simulink model "serial_plot_v1"  (R2019a)
settings: Solver=VariableStepAuto  StartTime=0.0  StopTime=inf  RelTol=1e-3
libraries: instrumentlib x2
settings Model: Creator=facuolmed_o  LastModifiedBy=facuolmed_o

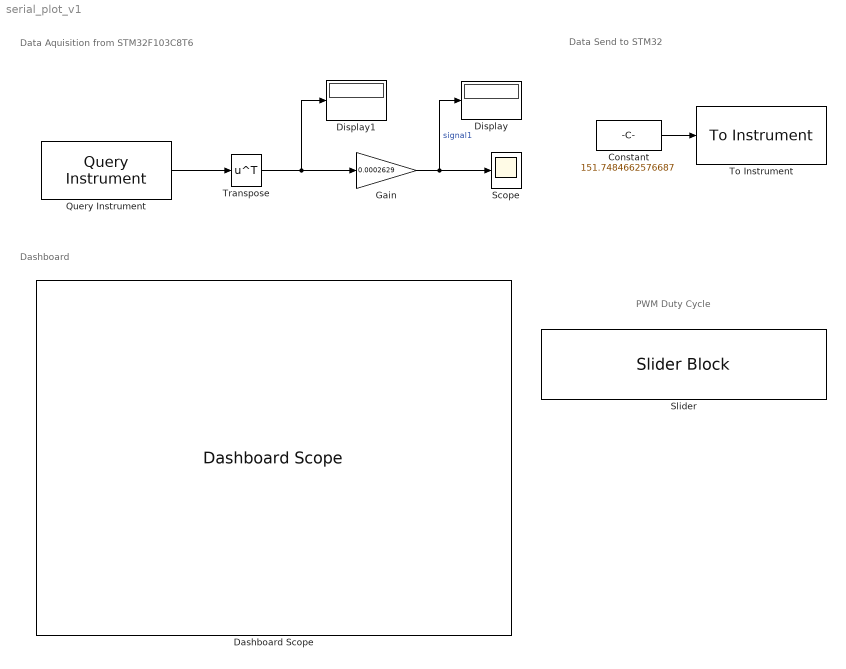
== system serial_plot_v1 ==
  note: PWM Duty Cycle
  note: Data Send to STM32
  note: Dashboard
  note: Data Aquisition from STM32F103C8T6
  Constant : Constant  Value=151.7484662576687  OutDataTypeStr=double  SampleTime=0
  Dashboard Scope : DashboardScope  TimeSpan=100  Ymin=-0.20000000000000001  Ymax=1.2
  Display : Display
      settings: Format=binary (Stored Integer)
  Display1 : Display
      settings: Format=bank
  Gain : Gain  Gain=0.0002629
  Query Instrument : instrumentlib/Query Instrument  sampleTime=0  isWorkspaceObject=off  timeout=10  inputBufferSize=512  protocol=Serial  serialPort=COM2  baudRate=115200  gpibVendor=Keysight Technologies  boardIndex=0  primaryAddress=1  secondaryAddress=0  visaVendor=Keysight  visaSerialPort=0  chassisIndex=0  logicalAddress=0  tcpRemoteHost='127.0.0.1'  tcpRemotePort=4500  udpRemoteHost='127.0.0.1'  udpRemotePort=9090  visaTCPBoardIndex=0  visaTCPRemoteHost='127.0.0.1'  usbBoardIndex=0  usbManufID=0  usbModelCode=0  usbSerialNumber=0  initAction=None  initCommand='DATA:SOURCE CH1'  initFunction=get  queryCommand=''  responseFormat=ASCII  asciiFormatting='%d,%d\n'  precision=8-bit unsigned integer  byteOrder=Little endian  valuesToRead=1  removeBytes=off  afterOutputAction=Repeat query for new data  enableFrames=on  frameSize=2
      settings: SourceProductName=Instrument Control Toolbox  SourceProductBaseCode=IC
  Scope : Scope
  Slider : SliderBlock  ScaleMax=255
  To Instrument : instrumentlib/To Instrument  sampleTime=0  isWorkspaceObject=off  timeout=10  inputBufferSize=100  protocol=Serial  serialPort=COM2  baudRate=115200  gpibVendor=ICS Electronics  boardIndex=0  primaryAddress=1  secondaryAddress=0  visaVendor=Keysight  visaSerialPort=0  chassisIndex=0  logicalAddress=0  tcpRemoteHost='127.0.0.1'  tcpRemotePort=4500  udpRemoteHost='127.0.0.1'  udpRemotePort=9090  visaTCPBoardIndex=0  visaTCPRemoteHost='127.0.0.1'  usbBoardIndex=0  usbManufID=0  usbModelCode=0  usbSerialNumber=0  initAction=None  initCommand='DATA:SOURCE CH1'  initFunction=get  command=''  sendFormat=Binary  asciiFormatting='%c'  precision=8-bit unsigned integer  byteOrder=Little endian
      settings: SourceProductName=Instrument Control Toolbox  SourceProductBaseCode=IC
  Transpose : Math  Operator=transpose  SaturateOnIntegerOverflow=on
  wires:
  Query Instrument/1 -> Transpose/1
  Gain/1 -> Scope/1, Display/1  "signal1"
  Transpose/1 -> Display1/1, Gain/1
  Constant/1 -> To Instrument/1
